simulink model "Modelo_controlador_integrador"  (R2021a)
settings: Solver=FixedStepAuto  StartTime=0.0  StopTime=38  FixedStep=0.001  RelTol=1e-3
libraries: simulink x1
settings Model: Creator=faust  LastModifiedBy=faust

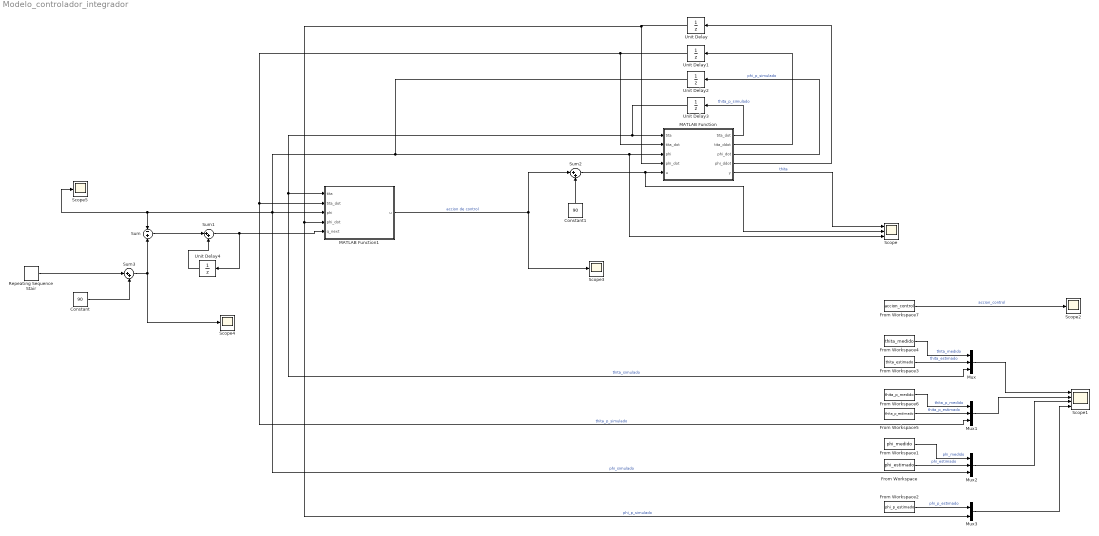
== system Modelo_controlador_integrador ==
  Constant : Constant  Value=90
  Constant1 : Constant  Value=90
  From Workspace : FromWorkspace  VariableName=phi_estimado
  From Workspace1 : FromWorkspace  VariableName=phi_medido
  From Workspace2 : FromWorkspace  VariableName=phi_p_estimado
  From Workspace3 : FromWorkspace  VariableName=thita_estimado
  From Workspace4 : FromWorkspace  VariableName=thita_medido
  From Workspace5 : FromWorkspace  VariableName=thita_p_estimado
  From Workspace6 : FromWorkspace  VariableName=thita_p_medido
  From Workspace7 : FromWorkspace  VariableName=accion_control
  MATLAB Function : MATLAB Function  TreatAsAtomicUnit=on
  MATLAB Function1 : MATLAB Function  TreatAsAtomicUnit=on
  Mux : Mux  Inputs=3
  Mux1 : Mux  Inputs=3
  Mux2 : Mux  Inputs=3
  Mux3 : Mux  Inputs=2
  Repeating Sequence Stair : simulink/Sources/Repeating Sequence Stair  OutValues=[0 10 -15 20 -25 30 -35]  tsamp=5  OutMin=[]  OutMax=[]  OutDataTypeStr=double  OutputDataTypeScalingMode=double  OutDataType=fixdt(0,8)  ConRadixGroup=Best Precision: Vector-wise  OutScaling=2^-12
  Scope : Scope  NumInputPorts=3
  Scope1 : Scope  NumInputPorts=4
  Scope{2..5} (4 alike) : Scope
  Sum : Sum  Inputs=-|+
  Sum1 : Sum  Inputs=|++
  Sum2 : Sum  Inputs=|++
  Sum3 : Sum  Inputs=|++
  Unit Delay{,1,3..4} (4 alike) : UnitDelay  SampleTime=0.01  HasFrameUpgradeWarning=on
  Unit Delay2 : UnitDelay  InitialCondition=90  SampleTime=0.01  HasFrameUpgradeWarning=on
  wires:
  MATLAB Function/2(tita_ddot) -> Unit Delay1/1
  Unit Delay1/1 -> MATLAB Function1/2(tita_dot), Mux1/3, MATLAB Function/2("tita_dot ")  "thita_p_simulado"
  MATLAB Function/5(y) -> Scope/1  "thita"
  MATLAB Function/4(phi_ddot) -> Unit Delay/1
  Unit Delay/1 -> Mux3/2, MATLAB Function1/4(phi_dot), MATLAB Function/4("phi_dot ")  "phi_p_simulado"
  MATLAB Function/3(phi_dot) -> Unit Delay2/1  "phi_p_simulado"
  MATLAB Function1/1(u) -> Sum2/1, Scope3/1  "accion de control"
  Constant1/1 -> Sum2/2
  From Workspace2/1 -> Mux3/1  "phi_p_estimado"
  From Workspace/1 -> Mux2/2  "phi_estimado"
  From Workspace6/1 -> Mux1/1  "thita_p_medido"
  Mux2/1 -> Scope1/3
  From Workspace1/1 -> Mux2/1  "phi_medido"
  Mux1/1 -> Scope1/2
  Mux/1 -> Scope1/1
  From Workspace3/1 -> Mux/2  "thita_estimado"
  From Workspace5/1 -> Mux1/2  "thita_p_estimado"
  From Workspace4/1 -> Mux/1  "thita_medido"
  Unit Delay3/1 -> MATLAB Function1/1(tita), Mux/3, MATLAB Function/1(tita)  "thita_simulado"
  Mux3/1 -> Scope1/4
  Unit Delay2/1 -> Scope/3, MATLAB Function/3(phi), Mux2/3, Sum/1, Scope5/1, MATLAB Function1/3(phi)  "phi_simulado"
  From Workspace7/1 -> Scope2/1  "accion_control"
  Sum2/1 -> Scope/2, MATLAB Function/5(u)
  MATLAB Function/1(tita_dot) -> Unit Delay3/1  "thita_p_simulado"
  Repeating Sequence Stair/1 -> Sum3/1
  Sum/1 -> Sum1/1
  Sum1/1 -> Unit Delay4/1, MATLAB Function1/5(q_next)
  Sum3/1 -> Sum/2, Scope4/1
  Constant/1 -> Sum3/2
  Unit Delay4/1 -> Sum1/2

== matlab function Modelo_controlador_integrador/MATLAB Function1 ==
  data: tita input; tita_dot input; phi input; u output; phi_dot input; q_next input
function u = fcn(tita, tita_dot,phi,phi_dot,q_next)

K = [-0.6891  ,  0.0954  ,  0.0943 ,  -0.0581  ,  0.0186];
phi_eq = 90;
u = K(1) * tita + K(2) * tita_dot + K(3) * (phi - phi_eq) + K(4) * phi_dot + K(5) * q_next;

== matlab function Modelo_controlador_integrador/MATLAB Function ==
  data: tita input; tita_dot input; tita_dot output; tita_ddot output; phi_dot output; phi input; phi_dot input; phi_ddot output; u input; y output
function [tita_dot, tita_ddot, phi_dot, phi_ddot, y] = fcn(tita, tita_dot, phi, phi_dot, u)

Ad = [
    1.0000    0.0100         0         0;
   -0.6500    0.9739   -2.0454   -0.2147;
         0         0    1.0000    0.0100;
         0         0   -2.9220    0.6933
];

Bd = [
         0;
    2.0454;
         0;
    2.9220
];

x  = [tita tita_dot phi phi_dot];
x_dot = Ad * x' + Bd * u;
tita_dot = x_dot(1);
tita_ddot = x_dot(2);
phi_dot = x_dot(3);
phi_ddot = x_dot(4);


y = x(1);
